simulink model "MAS_Full_State"  (R2021b)
settings: Solver=VariableStepAuto  StartTime=0.0  StopTime=10  RelTol=1e-3
libraries: cstblocks x15
settings Model: Creator=lenovo  LastModifiedBy=lenovo

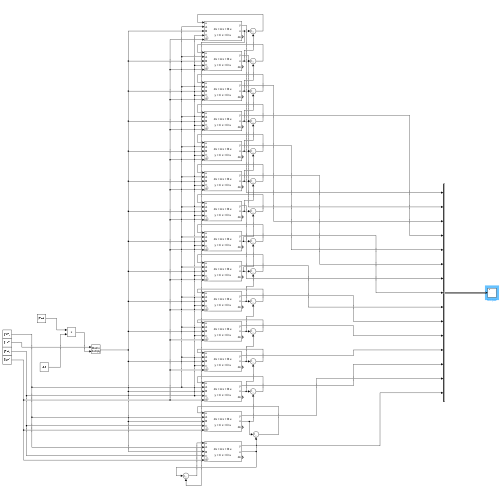
[thumbnail: Simulink's stored preview of the top-level diagram]
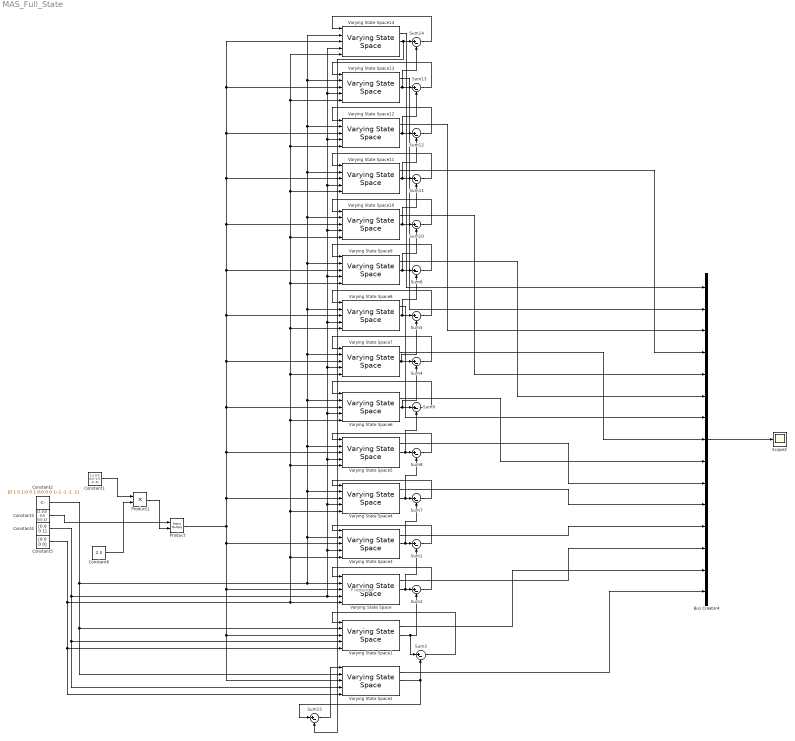
== system MAS_Full_State ==
  note: P resburger
  Bus Creator4 : BusCreator  Inputs=15
  Constant1 : Constant  Value=[-1 0 0 0;0 -1.5 -2 -1]
  Constant2 : Constant  Value=[0 1 0 1;0 0 1 0;0 0 0 1;-1 -1 -1 -1]
  Constant3 : Constant  Value=[1 0;0 0;0 0;0 1]
  Constant4 : Constant  Value=[0 0 0 1]  VectorParams1D=off
  Constant5 : Constant  Value=[0 0 0 0]  VectorParams1D=off
  Constant6 : Constant  Value=2.5  VectorParams1D=off
  Product : Product  Multiplication=Matrix(*)
  Product1 : Product
  Scope2 : Scope
  Sum{1..15} (15 alike) : Sum  Inputs=|+-
  Varying State Space{,1,3..14} (14 alike) : cstblocks/Linear Parameter Varying/Varying State Space  x0=0  xNames=''  OutputX=on  OutputDX=on
  Varying State Space2 : cstblocks/Linear Parameter Varying/Varying State Space  x0=[1;0;0;0]  xNames=''  OutputX=on  OutputDX=on
  wires:
  Constant2/1 -> Varying State Space2/2, Varying State Space1/2, Varying State Space3/2, Varying State Space4/2, Varying State Space5/2, Varying State Space7/2, Varying State Space8/2, Varying State Space9/2, Varying State Space10/2, Varying State Space11/2, Varying State Space12/2, Varying State Space14/2, Varying State Space13/2, Varying State Space6/2, Varying State Space/2
  Constant4/1 -> Varying State Space2/4, Varying State Space1/4, Varying State Space9/4, Varying State Space14/4, Varying State Space13/4, Varying State Space12/4, Varying State Space11/4, Varying State Space10/4, Varying State Space8/4, Varying State Space7/4, Varying State Space6/4, Varying State Space5/4, Varying State Space4/4, Varying State Space3/4, Varying State Space/4
  Constant5/1 -> Varying State Space2/5, Varying State Space1/5, Varying State Space3/5, Varying State Space4/5, Varying State Space5/5, Varying State Space7/5, Varying State Space8/5, Varying State Space9/5, Varying State Space10/5, Varying State Space11/5, Varying State Space13/5, Varying State Space14/5, Varying State Space12/5, Varying State Space6/5, Varying State Space/5
  Bus Creator4/1 -> Scope2/1
  Varying State Space1/2 -> Sum2/2, Sum3/1
  Constant3/1 -> Product/1
  Constant6/1 -> Product1/2
  Product/1 -> Varying State Space3/3, Varying State Space2/3, Varying State Space1/3, Varying State Space/3, Varying State Space7/3, Varying State Space8/3, Varying State Space9/3, Varying State Space10/3, Varying State Space11/3, Varying State Space12/3, Varying State Space14/3, Varying State Space13/3, Varying State Space6/3, Varying State Space5/3, Varying State Space4/3
  Varying State Space2/2 -> Sum15/1, Sum3/2
  Varying State Space/2 -> Sum1/2, Sum2/1
  Constant1/1 -> Product1/1
  Product1/1 -> Product/2
  Sum2/1 -> Varying State Space/1
  Sum3/1 -> Varying State Space1/1
  Varying State Space3/2 -> Sum7/2, Sum1/1
  Varying State Space4/2 -> Sum8/2, Sum7/1
  Varying State Space5/2 -> Sum9/2, Sum8/1
  Varying State Space6/2 -> Sum4/2, Sum9/1
  Sum1/1 -> Varying State Space3/1
  Sum7/1 -> Varying State Space4/1
  Sum8/1 -> Varying State Space5/1
  Sum9/1 -> Varying State Space6/1
  Varying State Space6/1 -> Bus Creator4/9
  Varying State Space5/1 -> Bus Creator4/10
  Varying State Space4/1 -> Bus Creator4/11
  Varying State Space3/1 -> Bus Creator4/12
  Varying State Space/1 -> Bus Creator4/13
  Varying State Space1/1 -> Bus Creator4/14
  Varying State Space2/1 -> Bus Creator4/15
  Sum4/1 -> Varying State Space7/1
  Varying State Space8/2 -> Sum6/2, Sum5/1
  Sum5/1 -> Varying State Space8/1
  Varying State Space9/2 -> Sum10/2, Sum6/1
  Sum6/1 -> Varying State Space9/1
  Varying State Space10/2 -> Sum11/2, Sum10/1
  Sum10/1 -> Varying State Space10/1
  Varying State Space11/2 -> Sum12/2, Sum11/1
  Sum11/1 -> Varying State Space11/1
  Varying State Space12/2 -> Sum13/2, Sum12/1
  Sum12/1 -> Varying State Space12/1
  Varying State Space13/2 -> Sum14/2, Sum13/1
  Sum13/1 -> Varying State Space13/1
  Sum14/1 -> Varying State Space14/1
  Varying State Space7/1 -> Bus Creator4/8
  Varying State Space8/1 -> Bus Creator4/7
  Varying State Space9/1 -> Bus Creator4/6
  Varying State Space10/1 -> Bus Creator4/5
  Varying State Space11/1 -> Bus Creator4/4
  Varying State Space12/1 -> Bus Creator4/3
  Varying State Space13/1 -> Bus Creator4/2
  Varying State Space14/1 -> Bus Creator4/1
  Varying State Space7/2 -> Sum5/2, Sum4/1
  Sum15/1 -> Varying State Space2/1
  Varying State Space14/2 -> Sum15/2, Sum14/1
